simulink model "feedbackTuning"  (R2016b)
settings: Solver=VariableStepAuto  StartTime=0.0  StopTime=0.6  RelTol=1e-3
values from neighbouring files (symbols this model uses):
  denGp = [m1*m2 0 (m1+m2)*k 0 0]    [mainFeedbackTuning.m]
  denominator = denominator{1}    [mainFeedbackTuning.m]
  m1 = 20    [mainFeedbackTuning.m]
  m2 = 5    [mainFeedbackTuning.m]
  numerator = numerator{1}    [mainFeedbackTuning.m]
  numGp = k    (= 6316546.8167)    [mainFeedbackTuning.m]
  Ts = 1/fs    (= 0.0001)    [mainFeedbackTuning.m]
  varNoise = sigma*sigma    (= 0)    [mainFeedbackTuning.m]
libraries: simulink x1, model_controller x1
settings Model: Creator=Dai Luyao  LastModifiedBy=Dai Luyao

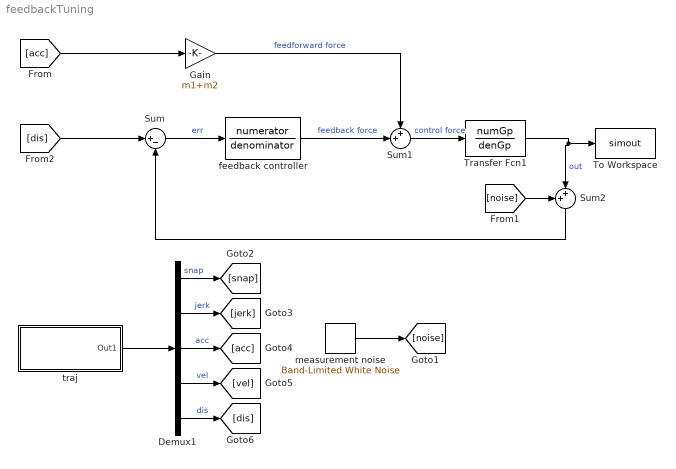
== system feedbackTuning ==
  Demux1 : Demux  Outputs=5
  Gain : Gain  Gain=m1+m2
  Sum : Sum  Inputs=|+-
  Sum1 : Sum  Inputs=++|
  Sum2 : Sum  Inputs=++|
  To Workspace : ToWorkspace  VariableName=simout  SampleTime=-1
  Transfer Fcn1 : TransferFcn  Numerator=numGp  Denominator=denGp
  feedback controller : TransferFcn  Numerator=numerator  Denominator=denominator
  measurement noise : simulink/Sources/Band-Limited White Noise  Cov=[varNoise*Ts]  Ts=Ts  seed=[23341]
  traj : Subsystem  BlockChoice=2th order traj
      settings: AttributesFormatString=%<BlockChoice>  TemplateBlock=model_controller/Profile Generators/traj  MemberBlocks=2th order traj,3rd order traj,4th order traj,step
  wires:
  Transfer Fcn1/1 -> Sum2/2, To Workspace/1  "out"
  Demux1/1 -> [snap]  "snap"
  Demux1/2 -> [jerk]  "jerk"
  Demux1/3 -> [acc]  "acc"
  Demux1/4 -> [vel]  "vel"
  Demux1/5 -> [dis]  "dis"
  Sum1/1 -> Transfer Fcn1/1  "control force"
  feedback controller/1 -> Sum1/2  "feedback force"
  Sum/1 -> feedback controller/1  "err"
  Gain/1 -> Sum1/1  "feedforward force"
  [dis] -> Sum/1
  [acc] -> Gain/1
  traj/1(Out1) -> Demux1/1
  measurement noise/1 -> [noise]
  [noise] -> Sum2/1
  Sum2/1 -> Sum/2

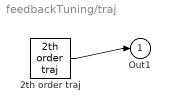
== system feedbackTuning/traj ==
  2th order traj : model_controller/Profile Generators/2th order traj  t0=0  x=0.06  v=0.25  a=10  Ts=0
  Out1 : Outport
  wires:
  2th order traj/1 -> Out1/1
